simulink model "OAC_LA_Ass1_Task3_linearization"  (R2018a)
settings: Solver=VariableStepAuto  StartTime=0.0  StopTime=10.0  MaxStep=1e-3  RelTol=1e-3
values from neighbouring files (symbols this model uses):
  all_params = [l, ms, mw, V, k1]    [OAC_LA_Ass1.m]
  g = 9.81    [OAC_LA_Ass1.m]
  x0 = [0, deg2rad(5), 0, 0]'    [OAC_LA_Ass1.m]
settings Model: Creator=lukastotschnig  LastModifiedBy=miko2

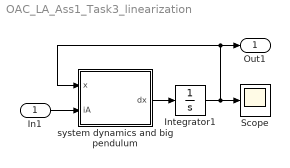
== system OAC_LA_Ass1_Task3_linearization ==
  In1 : Inport
  Integrator1 : Integrator  InitialCondition=x0
  Scope : Scope
  system dynamics and big pendulum : MATLAB Function  TreatAsAtomicUnit=on
  Out1 : Outport
  wires:
  system dynamics and big pendulum/1(dx) -> Integrator1/1
  Integrator1/1 -> system dynamics and big pendulum/1(x), Out1/1, Scope/1
  In1/1 -> system dynamics and big pendulum/2(iA)

== matlab function OAC_LA_Ass1_Task3_linearization/system dynamics and big pendulum ==
  data: dx output; x input; iA input; all_params parameter; g parameter
function dx  = fcn(x,iA,all_params,g)
    
    l = all_params(1);
    ms = all_params(2);
    mw = all_params(3);
    V = all_params(4);
    k1 = all_params(5);
    
    
    x_W = x(1);
    phi = x(2);
    v_W = x(3);
    omega = x(4);
    
    F = V*iA - k1*v_W;

    dx_W = v_W;
    dphi = omega;
    dv_W = 1/( mw + ms*(1-(cos(phi))^2) ) * ( F + ms*l*omega^2*sin(phi) ...
        - ms*g*sin(phi)*cos(phi) );
    domega = 1/( l * ( 1 - ms/(mw+ms)*(cos(phi))^2 ) ) * ( g*sin(phi) - ...
        cos(phi)/(ms+mw)*F - ms/(mw+ms)*l*omega^2*sin(phi)*cos(phi) );
    
    dx = [dx_W; dphi; dv_W; domega]; 

end
